simulink library "libMdl_AttitudeComputer"  (R2019b)
settings: Solver=VariableStepAuto  StartTime=0.0  StopTime=10.0  RelTol=1e-3
undefined symbols (not defined in the file): comp_filter_adaptive_gain_thresholds, comp_filter_static_gain, sample_time
libraries: libMdl_transformVect x2, libMdl_multQuat x1, simulink x1, libMdl_invQuat x1
settings Model: Creator=Hanno  LastModifiedBy=Hanno

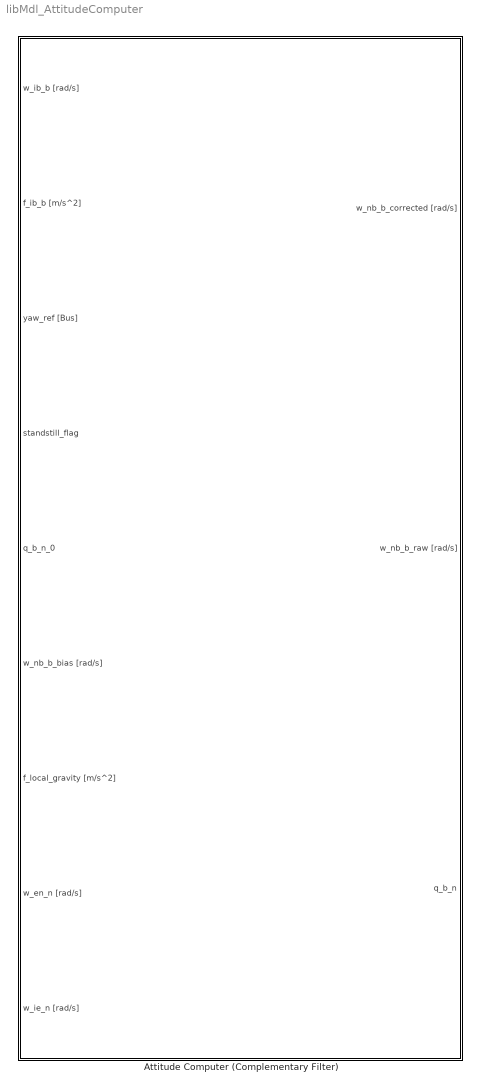
== system libMdl_AttitudeComputer ==
  Attitude Computer (Complementary Filter) : Subsystem  mask(Attitude Computer){mv_static_alpha=comp_filter_static_gain, mv_adaptive_gain_thresholds=comp_filter_adaptive_gain_thresholds, mv_enable_heading_correction=on, mv_sample_time=-1}
      mask prompts: mv_static_alpha "Static Alpha:"; mv_adaptive_gain_thresholds "Adaptive Gain Thresholds:"; mv_enable_heading_correction "Enable Heading Correction:"; mv_sample_time "Sample Time [s]:"
      mask help:
      | Attitude computer utilizing the complementary filter presented from Valenti et al.
      |
      | See:
      | - Valenti et al., "Keeping a Good Attitude: A Quaternion-Based Orientation Filter for IMUs and MARGs", Sensors, pp. 19302-19330, 2015
      | - D. Titterton and J. Westen, "Strapdown Inertial Navigation Technology", IET, 2004
      settings: AttributesFormatString="see: Valenti et al., \"Keeping a Good Attitude: A Quaternion-Based Orientation Filter for IMUs and MARGs\", Sensors, pp. 19302-19330, 2015"
      mask DialogControl ParameterGroupVar Prompt: Complementary Filter Parameters
      mask Display:
      | if mv_enable_heading_correction
      |     heading_str = 'on';
      | else
      |     heading_str = 'off';
      | end % if
      | 
      | str1 = sprintf('\\color{black}{\\bfAttitude Calculation}\n\n');
      | str2 = sprintf('Static Alpha: %0.3f\n',mv_static_alpha);
      | str3 = sprintf('Adaptive Gain Thresholds: [%0.3f %0.3f]\n',mv_adaptive_gain_thresholds(1),mv_adaptive_gain_thresholds(2));
      | str4 = sprintf('Enable Heading Correction: %s\n',heading_str);
      | str5 = sprintf('Sample Time: %0.3f',mv_sample_time);
      | 
      | str = [str1,str2,str3,str4,str5];
      | 
      | text( 0.5,0.5, ...
      |       str, ...
      |       'horizontalAlignment', 'center', ...
      |       'texmode','on' ...
      |     )

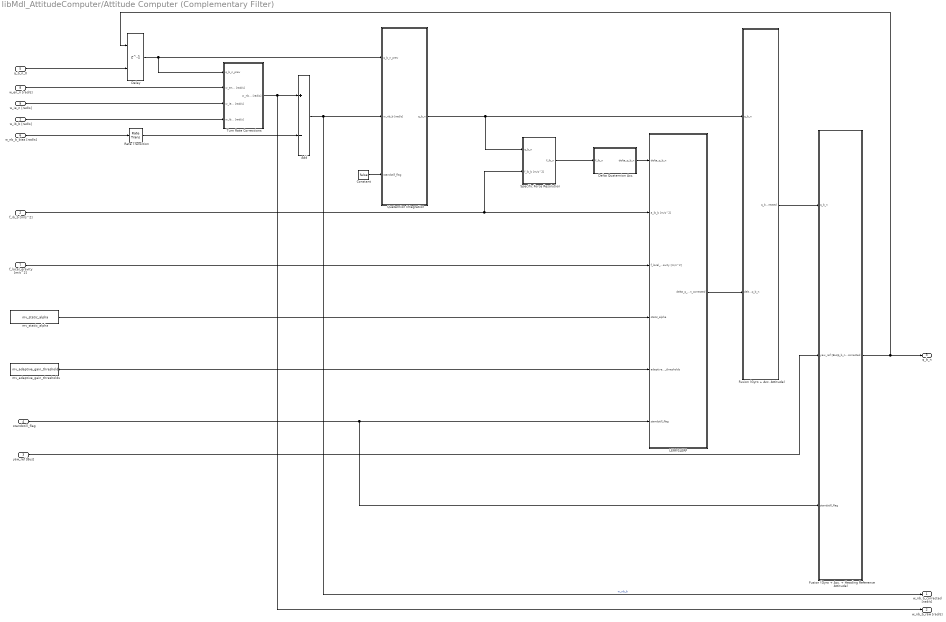
== system libMdl_AttitudeComputer/Attitude Computer (Complementary Filter) ==
  w_ib_b [rad/s] : Inport
  f_ib_b [m/s^2] : Inport  Port=2
  yaw_ref [Bus] : Inport  Port=3
  standstill_flag : Inport  Port=4
  q_b_n_0 : Inport  Port=5
  w_nb_b_bias [rad/s] : Inport  Port=6
  f_local_gravity [m/s^2] : Inport  Port=7
  w_en_n [rad/s] : Inport  Port=8
  w_ie_n [rad/s] : Inport  Port=9
  Add : Sum  Inputs=+-
  Constant : Constant  Value=false
  Delay : Delay  DelayLength=1  InitialConditionSource=Input port
      settings: InputPortMap=u0,p4
  Delta Quaternion Acc. : Subsystem
  Fusion (Gyro + Acc. + Heading Reference Attitude) : Subsystem
  Fusion (Gyro + Acc. Attitude) : Subsystem
  LERP/SLERP : Subsystem
  Quaternion Integration : Subsystem
      settings: AttributesFormatString="See:  D. Titterton and J. Westen, \"Strapdown Inertial Navigation Technology\", pp. 319-320, IET, 2004"
  Rate Transition : RateTransition  OutPortSampleTime=mv_sample_time
  Specific Force Resolution : Subsystem
  Turn Rate Corrections : Subsystem  TreatAsAtomicUnit=on  SystemSampleTime=mv_sample_time
  mv_adaptive_gain_thresholds : Constant  Value=mv_adaptive_gain_thresholds
  mv_static_alpha : Constant  Value=mv_static_alpha
  w_nb_b_corrected [rad/s] : Outport  VectorParamsAs1DForOutWhenUnconnected=off
  w_nb_b_raw [rad/s] : Outport  Port=2  VectorParamsAs1DForOutWhenUnconnected=off
  q_b_n : Outport  Port=3  VectorParamsAs1DForOutWhenUnconnected=off
  wires:
  Rate Transition/1 -> Add/2
  yaw_ref [Bus]/1 -> Fusion (Gyro + Acc. + Heading Reference Attitude)/2(yaw_ref [Bus])
  Constant/1 -> Quaternion Integration/3(standstill_flag)
  mv_adaptive_gain_thresholds/1 -> LERP/SLERP/5(adaptive_gain_thresholds)
  standstill_flag/1 -> LERP/SLERP/6(standstill_flag), Fusion (Gyro + Acc. + Heading Reference Attitude)/3(standstill_flag)
  f_local_gravity [m/s^2]/1 -> LERP/SLERP/3(f_local_gravity [m/s^2])
  mv_static_alpha/1 -> LERP/SLERP/4(static_alpha)
  q_b_n_0/1 -> Delay/2
  LERP/SLERP/1(delta_q_b_n_corrected) -> Fusion (Gyro + Acc. Attitude)/2(delta_q_b_n)
  Quaternion Integration/1(q_b_n) -> Fusion (Gyro + Acc. Attitude)/1(q_b_n), Specific Force Resolution/1(q_b_n)
  Fusion (Gyro + Acc. + Heading Reference Attitude)/1(q_b_n_corrected) -> q_b_n/1, Delay/1
  Fusion (Gyro + Acc. Attitude)/1(q_b_n_corrected) -> Fusion (Gyro + Acc. + Heading Reference Attitude)/1(q_b_n)
  Delta Quaternion Acc./1(delta_q_b_n) -> LERP/SLERP/1(delta_q_b_n)
  f_ib_b [m/s^2]/1 -> LERP/SLERP/2(a_ib_b [m/s^2]), Specific Force Resolution/2(f_ib_b [m/s^2])
  w_ie_n [rad/s]/1 -> Turn Rate Corrections/3(w_ie_n [rad/s])
  w_en_n [rad/s]/1 -> Turn Rate Corrections/2(w_en_n [rad/s])
  w_ib_b [rad/s]/1 -> Turn Rate Corrections/4(w_ib_b [rad/s])
  Delay/1 -> Quaternion Integration/1(q_b_n_prev), Turn Rate Corrections/1(q_b_n_prev)
  w_nb_b_bias [rad/s]/1 -> Rate Transition/1
  Turn Rate Corrections/1(w_nb_b [rad/s]) -> w_nb_b_raw [rad/s]/1, Add/1
  Specific Force Resolution/1(f_ib_n) -> Delta Quaternion Acc./1(f_ib_n)
  Add/1 -> Quaternion Integration/2(w_nb_b [rad/s]), w_nb_b_corrected [rad/s]/1  "w_nb_b"

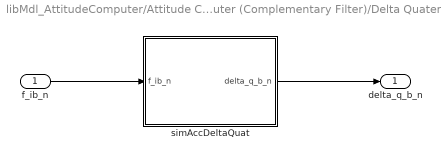
== system libMdl_AttitudeComputer/Attitude Computer (Complementary Filter)/Delta Quaternion Acc. ==
  f_ib_n : Inport
  simAccDeltaQuat : MATLAB Function  TreatAsAtomicUnit=on
  delta_q_b_n : Outport  VectorParamsAs1DForOutWhenUnconnected=off
  wires:
  simAccDeltaQuat/1(delta_q_b_n) -> delta_q_b_n/1
  f_ib_n/1 -> simAccDeltaQuat/1(f_ib_n)

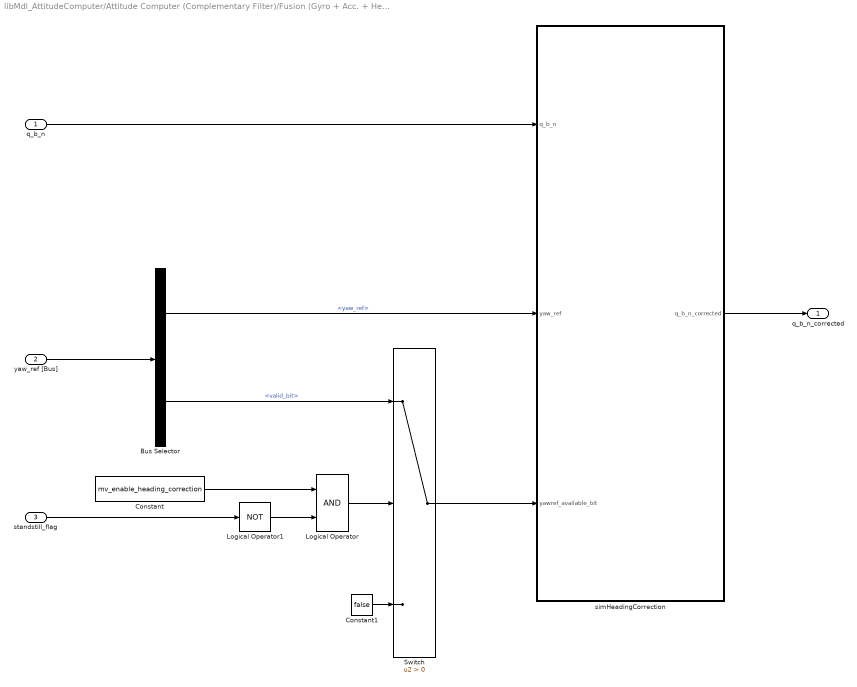
== system libMdl_AttitudeComputer/Attitude Computer (Complementary Filter)/Fusion (Gyro + Acc. + Heading Reference Attitude) ==
  q_b_n : Inport
  yaw_ref [Bus] : Inport  Port=2
  standstill_flag : Inport  Port=3
  Bus Selector : BusSelector  OutputSignals=yaw_ref,valid_bit
  Constant : Constant  Value=mv_enable_heading_correction
  Constant1 : Constant  Value=false
  Logical Operator : Logic  AllPortsSameDT=off  OutDataTypeStr=boolean
  Logical Operator1 : Logic  Operator=NOT  AllPortsSameDT=off  OutDataTypeStr=boolean
  Switch : Switch  Criteria=u2 > Threshold
  simHeadingCorrection : MATLAB Function  TreatAsAtomicUnit=on  SystemSampleTime=mv_sample_time
  q_b_n_corrected : Outport  VectorParamsAs1DForOutWhenUnconnected=off
  wires:
  standstill_flag/1 -> Logical Operator1/1
  Logical Operator1/1 -> Logical Operator/2
  Constant/1 -> Logical Operator/1
  Logical Operator/1 -> Switch/2
  Switch/1 -> simHeadingCorrection/3(yawref_available_bit)
  Constant1/1 -> Switch/3
  simHeadingCorrection/1(q_b_n_corrected) -> q_b_n_corrected/1
  q_b_n/1 -> simHeadingCorrection/1(q_b_n)
  yaw_ref [Bus]/1 -> Bus Selector/1
  Bus Selector/1 -> simHeadingCorrection/2(yaw_ref)  "<yaw_ref>"
  Bus Selector/2 -> Switch/1  "<valid_bit>"

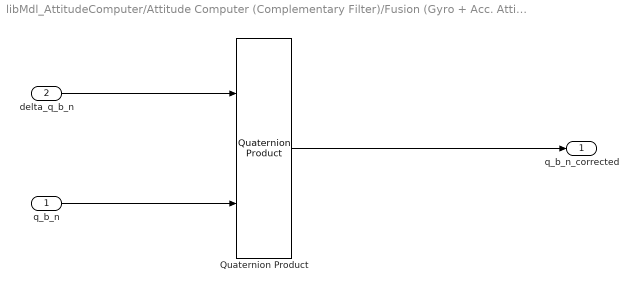
== system libMdl_AttitudeComputer/Attitude Computer (Complementary Filter)/Fusion (Gyro + Acc. Attitude) ==
  q_b_n : Inport
  delta_q_b_n : Inport  Port=2
  Quaternion Product : libMdl_multQuat/Quaternion Product  SystemSampleTime=-1  Latency=0  AutoFrameSizeCalculation=off
  q_b_n_corrected : Outport  VectorParamsAs1DForOutWhenUnconnected=off
  wires:
  Quaternion Product/1 -> q_b_n_corrected/1
  q_b_n/1 -> Quaternion Product/2
  delta_q_b_n/1 -> Quaternion Product/1

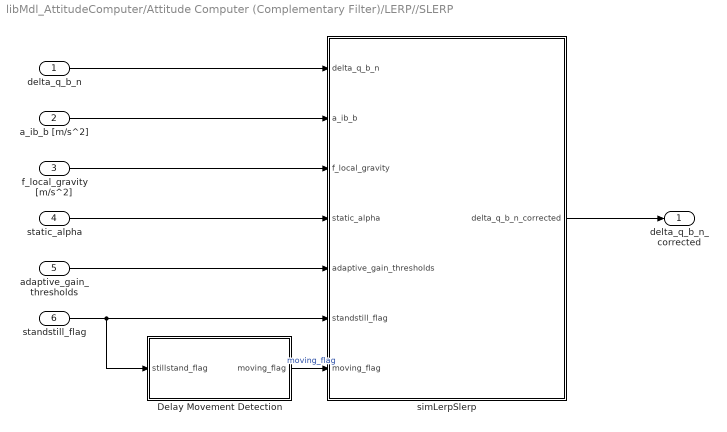
== system libMdl_AttitudeComputer/Attitude Computer (Complementary Filter)/LERP//SLERP ==
  delta_q_b_n : Inport
  a_ib_b [m/s^2] : Inport  Port=2
  f_local_gravity [m/s^2] : Inport  Port=3
  static_alpha : Inport  Port=4
  adaptive_gain_thresholds : Inport  Port=5
  standstill_flag : Inport  Port=6
  "Delay Movement Detection " : Subsystem  mask{mv_moving_detection_delay=0.2}
      mask prompts: mv_moving_detection_delay "Moving detection delay [s]:"
  simLerpSlerp : MATLAB Function  TreatAsAtomicUnit=on  SystemSampleTime=mv_sample_time
  delta_q_b_n_corrected : Outport  VectorParamsAs1DForOutWhenUnconnected=off
  wires:
  "Delay Movement Detection "/1(moving_flag) -> simLerpSlerp/7(moving_flag)  "moving_flag"
  delta_q_b_n/1 -> simLerpSlerp/1(delta_q_b_n)
  f_local_gravity [m/s^2]/1 -> simLerpSlerp/3(f_local_gravity)
  simLerpSlerp/1(delta_q_b_n_corrected) -> delta_q_b_n_corrected/1
  a_ib_b [m/s^2]/1 -> simLerpSlerp/2(a_ib_b)
  static_alpha/1 -> simLerpSlerp/4(static_alpha)
  adaptive_gain_thresholds/1 -> simLerpSlerp/5(adaptive_gain_thresholds)
  standstill_flag/1 -> simLerpSlerp/6(standstill_flag), "Delay Movement Detection "/1(stillstand_flag)

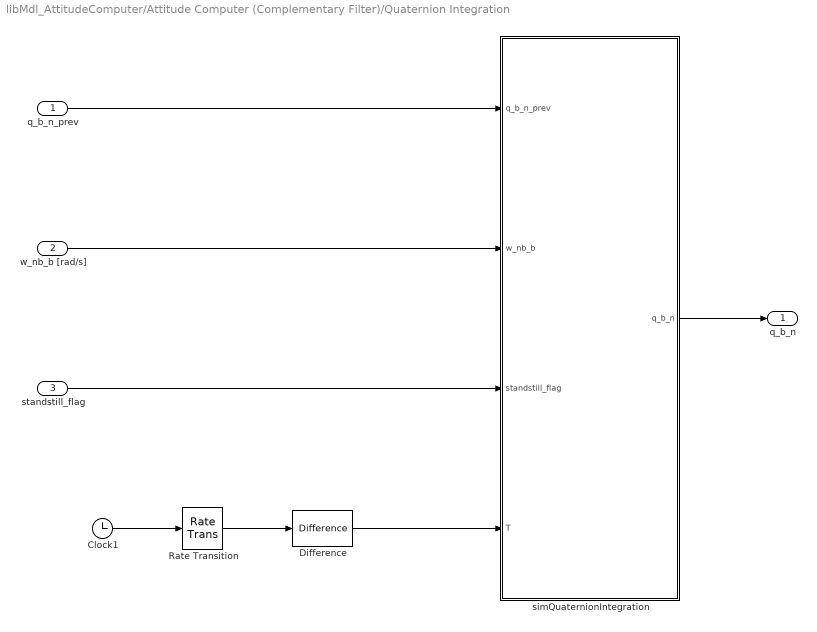
== system libMdl_AttitudeComputer/Attitude Computer (Complementary Filter)/Quaternion Integration ==
  q_b_n_prev : Inport
  w_nb_b [rad/s] : Inport  Port=2
  standstill_flag : Inport  Port=3
  Clock1 : Clock
  Difference : simulink/Discrete/Difference  ICPrevInput=0.0  OutMin=[]  OutMax=[]  OutDataType=fixdt(1, 16)  OutScaling=2^-10  DoSatur=off
  Rate Transition : RateTransition
  simQuaternionIntegration : MATLAB Function  TreatAsAtomicUnit=on  SystemSampleTime=mv_sample_time
  q_b_n : Outport  VectorParamsAs1DForOutWhenUnconnected=off
  wires:
  Rate Transition/1 -> Difference/1
  Clock1/1 -> Rate Transition/1
  simQuaternionIntegration/1(q_b_n) -> q_b_n/1
  q_b_n_prev/1 -> simQuaternionIntegration/1(q_b_n_prev)
  w_nb_b [rad/s]/1 -> simQuaternionIntegration/2(w_nb_b)
  standstill_flag/1 -> simQuaternionIntegration/3(standstill_flag)
  Difference/1 -> simQuaternionIntegration/4(T)

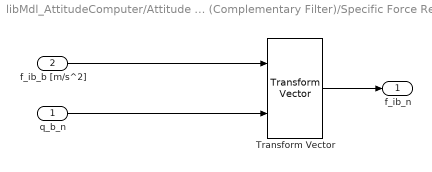
== system libMdl_AttitudeComputer/Attitude Computer (Complementary Filter)/Specific Force Resolution ==
  q_b_n : Inport
  f_ib_b [m/s^2] : Inport  Port=2
  Transform Vector : libMdl_transformVect/Transform Vector  SystemSampleTime=-1  Latency=0  AutoFrameSizeCalculation=off
  f_ib_n : Outport  VectorParamsAs1DForOutWhenUnconnected=off
  wires:
  f_ib_b [m/s^2]/1 -> Transform Vector/1
  Transform Vector/1 -> f_ib_n/1
  q_b_n/1 -> Transform Vector/2

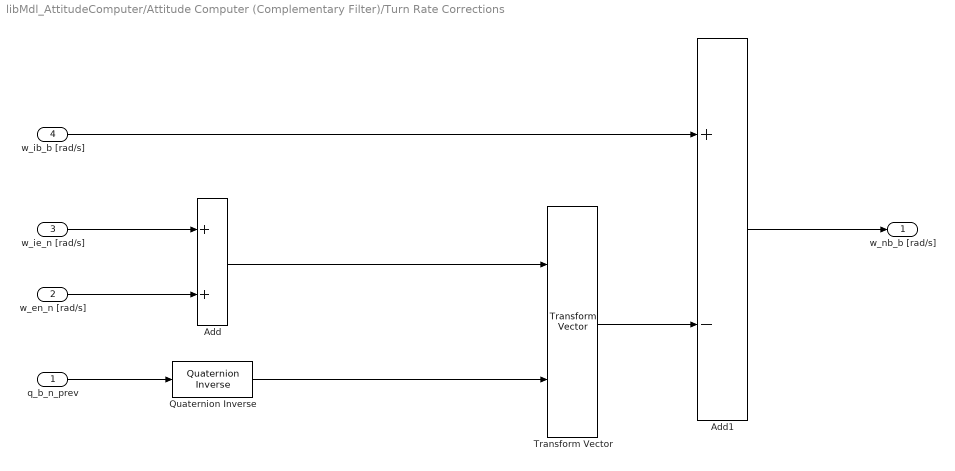
== system libMdl_AttitudeComputer/Attitude Computer (Complementary Filter)/Turn Rate Corrections ==
  q_b_n_prev : Inport
  w_en_n [rad/s] : Inport  Port=2
  w_ie_n [rad/s] : Inport  Port=3
  w_ib_b [rad/s] : Inport  Port=4
  Add : Sum
  Add1 : Sum  Inputs=+-
  Quaternion Inverse : libMdl_invQuat/Quaternion Inverse  SystemSampleTime=-1  Latency=0  AutoFrameSizeCalculation=off
  Transform Vector : libMdl_transformVect/Transform Vector  SystemSampleTime=-1  Latency=0  AutoFrameSizeCalculation=off
  w_nb_b [rad/s] : Outport  VectorParamsAs1DForOutWhenUnconnected=off
  wires:
  Quaternion Inverse/1 -> Transform Vector/2
  w_ie_n [rad/s]/1 -> Add/1
  w_en_n [rad/s]/1 -> Add/2
  Add/1 -> Transform Vector/1
  q_b_n_prev/1 -> Quaternion Inverse/1
  Transform Vector/1 -> Add1/2
  w_ib_b [rad/s]/1 -> Add1/1
  Add1/1 -> w_nb_b [rad/s]/1

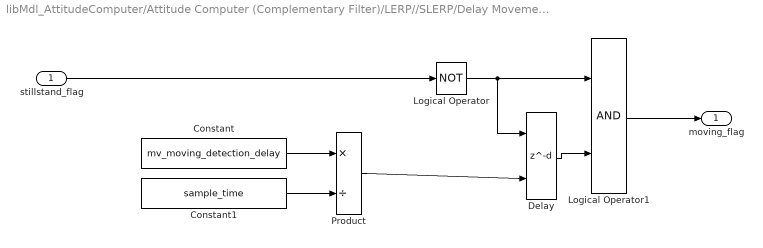
== system libMdl_AttitudeComputer/Attitude Computer (Complementary Filter)/LERP//SLERP/Delay Movement Detection  ==
  stillstand_flag : Inport
  Constant : Constant  Value=mv_moving_detection_delay
  Constant1 : Constant  Value=sample_time
  Delay : Delay  DelayLengthSource=Input port  DelayLength=0.1/sample_time
      settings: InputPortMap=u0,p1
  Logical Operator : Logic  Operator=NOT  AllPortsSameDT=off  OutDataTypeStr=boolean
  Logical Operator1 : Logic  AllPortsSameDT=off  OutDataTypeStr=boolean
  Product : Product  Inputs=*/
  moving_flag : Outport
  wires:
  Product/1 -> Delay/2
  Constant1/1 -> Product/2
  Constant/1 -> Product/1
  Logical Operator1/1 -> moving_flag/1
  stillstand_flag/1 -> Logical Operator/1
  Logical Operator/1 -> Logical Operator1/1, Delay/1
  Delay/1 -> Logical Operator1/2

== matlab function libMdl_AttitudeComputer/Attitude Computer (Complementary Filter)/Delta Quaternion Acc./simAccDeltaQuat ==
  data: f_ib_n input; delta_q_b_n output
function delta_q_b_n = simAccDeltaQuat(f_ib_n)

f_ib_n_ref = [0;0;-1];
delta_q_b_n = quatFromVect(f_ib_n,f_ib_n_ref);

end % function

== matlab function libMdl_AttitudeComputer/Attitude Computer (Complementary Filter)/Fusion (Gyro + Acc. + Heading Reference Attitude)/simHeadingCorrection ==
  data: q_b_n_corrected output; q_b_n input; yaw_ref input; yawref_available_bit input
function q_b_n_corrected = simHeadingCorrection(q_b_n,yaw_ref,yawref_available_bit)

if yawref_available_bit
    
    current_attitude = quatToEuler(q_b_n);    
    heading_diff = yaw_ref-current_attitude(3);
    
    if abs(heading_diff) < deg2rad(0.02)
        q_b_n_corrected = q_b_n;
    else
        q_correction = [cos(heading_diff/2);0;0;sin(heading_diff/2)];    
        q_b_n_corrected = multQuat(q_correction,q_b_n);
        %q_b_n_corrected = multQuat(q_b_v,multQuat(q_correction,q_b_n));
    end % if    
    
else
    
    q_b_n_corrected = q_b_n;
    %q_b_n_corrected = multQuat(q_b_v,q_b_n);
    
end % if

q_b_n_corrected = normalizeQuat(q_b_n_corrected);

end % function

== matlab function libMdl_AttitudeComputer/Attitude Computer (Complementary Filter)/LERP//SLERP/simLerpSlerp ==
  data: delta_q_b_n input; a_ib_b input; delta_q_b_n_corrected output; f_local_gravity input; static_alpha input; adaptive_gain_thresholds input; standstill_flag input; moving_flag input
function delta_q_b_n_corrected = fcn(delta_q_b_n,a_ib_b,f_local_gravity,static_alpha,adaptive_gain_thresholds,standstill_flag,moving_flag)

delta_q_b_n_corrected = delta_q_b_n;
q_I = [1;0;0;0];
epsilon = 0.9;

if standstill_flag 
    alpha = static_alpha;    
% elseif motion_flag    
%     alpha = 0;    
else
    adaptive_gain = calcGainFactor(a_ib_b,f_local_gravity,adaptive_gain_thresholds);
    alpha = static_alpha*adaptive_gain;
end % if

% SLERP    
if delta_q_b_n(1) < epsilon

    Omega = acos(delta_q_b_n(1));

    delta_q_b_n_corrected = sin((1-alpha)*Omega)/sin(Omega)*q_I + sin(alpha*Omega)/sin(Omega)*delta_q_b_n;
else % LERP

    delta_q_b_n_corrected = (1-alpha)*q_I + alpha*delta_q_b_n;       

end % if

% Normalization
delta_q_b_n_corrected = normalizeQuat(delta_q_b_n_corrected);

% if 0 == steady_state_flag
%     
%     delta_q_b_n_corrected = q_I;
% 
% else
%     
%     % SLERP    
%     if delta_q_b_n(1) < epsilon
% 
%         Omega = acos(delta_q_b_n(1));
% 
%         delta_q_b_n_corrected = sin((1-alpha)*Omega)/sin(Omega)*q_I + sin(alpha*Omega)/sin(Omega)*delta_q_b_n;
%     else % LERP
% 
%         delta_q_b_n_corrected = (1-alpha)*q_I + alpha*delta_q_b_n;       
% 
%     end % if
%     
%     % Normalization
%     delta_q_b_n_corrected = normalizeQuat(delta_q_b_n_corrected);
%     
% end % if

end % function

%% Helper Functions

function gain_factor = calcGainFactor(a_ib_b,f_local_gravity,adaptive_gain_thresholds)

a_norm = sqrt(sum(a_ib_b.^2));
g_norm = sqrt(sum(f_local_gravity.^2));
e = abs(a_norm-g_norm)/g_norm;

m = -1 / (adaptive_gain_thresholds(2)-adaptive_gain_thresholds(1));
n = 1-m*adaptive_gain_thresholds(1);

gain_factor = m*e+n;
gain_factor = min(max(gain_factor,0),1);

end % function

== matlab function libMdl_AttitudeComputer/Attitude Computer (Complementary Filter)/Quaternion Integration/simQuaternionIntegration ==
  data: q_b_n_prev input; w_nb_b input; standstill_flag input size=1; q_b_n output; T input
function q_b_n = fcn(q_b_n_prev,w_nb_b,standstill_flag,T)
% See:  D. Titterton and J. Westen, "Strapdown Inertial Navigation Technology", pp. 319-320, IET, 2004
%

if 0 == standstill_flag
    
    sigma = w_nb_b.*T;
    sigma_norm = sqrt(sum(sigma.^2));

    a_c = cos(sigma_norm/2);
    if sigma_norm > 1e-3
        a_s = sin(sigma_norm/2)/sigma_norm;
    else
        a_s = 0.5;
    end % if

    q_k = q_b_n_prev;
    r_k = [a_c;a_s.*sigma];
    q_k_new = multQuat(q_k,r_k);

    q_b_n = normalizeQuat(q_k_new);

else
   
    q_b_n = q_b_n_prev;
    
end % if

end % function
